simulink model "simulink"  (R2020a)
settings: Solver=ode1  StartTime=0.0  StopTime=StopTime  FixedStep=0.001  RelTol=1e-3
values from neighbouring files (symbols this model uses):
  Kd = ((K*M)/(600*Kt*omega_0))    [script.m]
  Kp = z*Kd    [script.m]
  Kt = 3.575e-05    [script.m]
  M = 1    [script.m]
  omega_0 = sqrt(G*M/Kt)    [script.m]
  Z0 = 2    [script.m]
  Zref = 1    [script.m]
settings Model: Creator=augus  LastModifiedBy=augus
settings DebuggingCC: UnconnectedInputMsg=none  UnconnectedOutputMsg=none  UnconnectedLineMsg=none  SFMachineParentedDataDiag=error

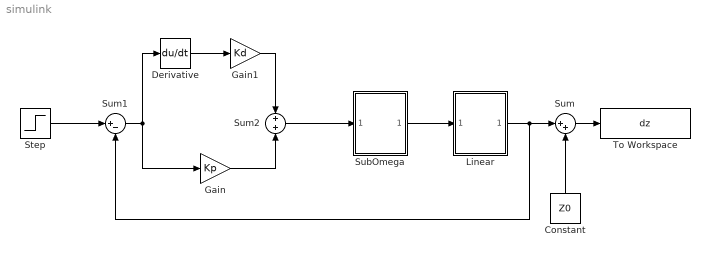
== system simulink ==
  Constant : Constant  Value=Z0
  Derivative : Derivative
  Gain : Gain  Gain=Kp
  Gain1 : Gain  Gain=Kd
  Linear : Subsystem
  Step : Step  After=Zref  SampleTime=0
  SubOmega : Subsystem
  Sum : Sum  Inputs=|++
  Sum1 : Sum  Inputs=|+-
  Sum2 : Sum
  To Workspace : ToWorkspace  VariableName=dz  SaveFormat=Structure With Time  SampleTime=-1
  wires:
  Constant/1 -> Sum/2
  SubOmega/1(δω(t)) -> Linear/1(δω(t))
  Sum/1 -> To Workspace/1
  Step/1 -> Sum1/1
  Linear/1(δz(t)) -> Sum1/2, Sum/1
  Sum1/1 -> Derivative/1, Gain/1
  Derivative/1 -> Gain1/1
  Gain1/1 -> Sum2/1
  Gain/1 -> Sum2/2
  Sum2/1 -> SubOmega/1(δu(t))

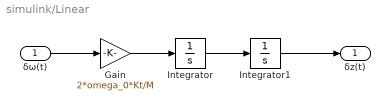
== system simulink/Linear ==
  δω(t) : Inport
  Gain : Gain  Gain=2*omega_0*Kt/M
  Integrator : Integrator
  Integrator1 : Integrator
  δz(t) : Outport
  wires:
  Integrator/1 -> Integrator1/1
  Gain/1 -> Integrator/1
  Integrator1/1 -> δz(t)/1
  δω(t)/1 -> Gain/1

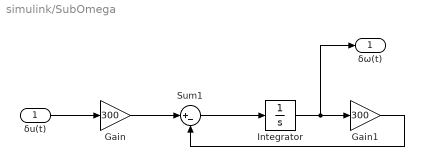
== system simulink/SubOmega ==
  δu(t) : Inport
  Gain : Gain  Gain=300
  Gain1 : Gain  Gain=300
  Integrator : Integrator
  Sum1 : Sum  Inputs=|+-
  δω(t) : Outport
  wires:
  Sum1/1 -> Integrator/1
  Gain/1 -> Sum1/1
  Integrator/1 -> δω(t)/1, Gain1/1
  Gain1/1 -> Sum1/2
  δu(t)/1 -> Gain/1
